simulink model "masseRessort"  (R2014b)
settings: Solver=ode45  StartTime=t0  StopTime=tf  MaxStep=max_step  MinStep=min_step  RelTol=tol
StopFcn:
  | save(wSaveFileName,wSwitchOutputName,wMatlabOutputName)
values from neighbouring files (symbols this model uses):
  b = bs(j)    [masseRessortDataDictionnary.m]    (also in masseRessortDataPost.m)
  b2 = 0    [masseRessortDataDictionnary.m]
  g = 9.8    [masseRessortDataDictionnary.m]
  k1 = 1    [masseRessortDataDictionnary.m]
  k2 = k2s(i)    [masseRessortDataDictionnary.m]    (also in masseRessortDataPost.m)
  m = 1    [masseRessortDataDictionnary.m]
  v0 = -3    [masseRessortDataDictionnary.m]
  x0 = 2    [masseRessortDataDictionnary.m]
  x1 = 1    [masseRessortDataDictionnary.m]
settings Model: Creator=Zangdaarr  LastModifiedBy=Zangdaarr
settings OptimizationCC: InlineParams=on  InlineInvariantSignals=on  EfficientFloat2IntCast=on

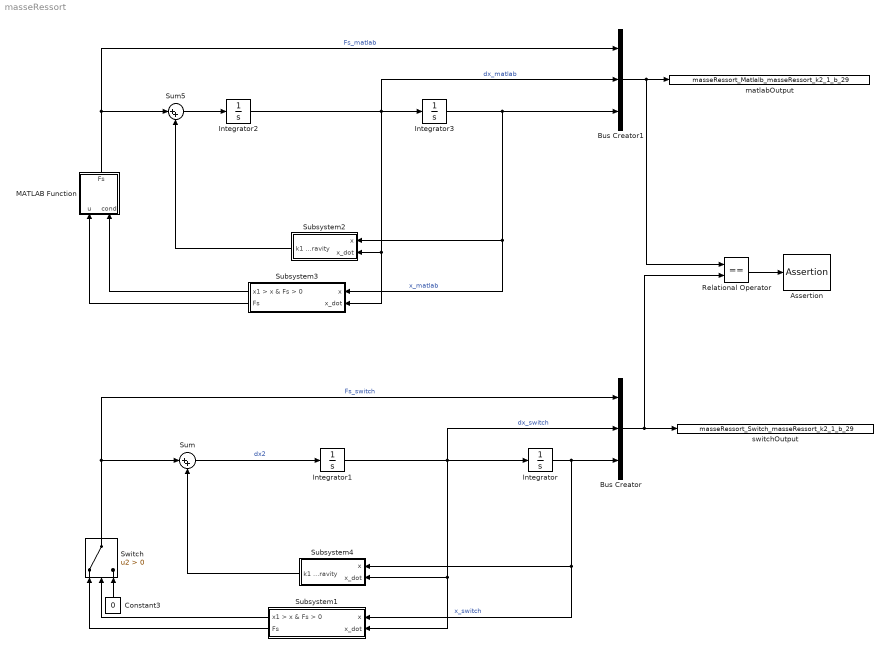
== system masseRessort ==
  Assertion : Assertion
  Bus Creator : BusCreator  Inputs=3
  Bus Creator1 : BusCreator  Inputs=3
  Constant3 : Constant  Value=0
  Integrator : Integrator  InitialCondition=x0
  Integrator1 : Integrator  InitialCondition=v0
  Integrator2 : Integrator  InitialCondition=v0
  Integrator3 : Integrator  InitialCondition=x0
  MATLAB Function : MATLAB Function  TreatAsAtomicUnit=on
  Relational Operator : RelationalOperator  Operator===  OutDataTypeStr=boolean
  Subsystem1 : Subsystem
  Subsystem2 : Subsystem
  Subsystem3 : Subsystem
  Subsystem4 : Subsystem
  Sum : Sum  Inputs=|++
  Sum5 : Sum  Inputs=|++
  Switch : Switch  Criteria=u2 > Threshold
  matlabOutput : ToWorkspace  VariableName=masseRessort_Matlalb_masseRessort_k2_1_b_29  SaveFormat=Timeseries  SampleTime=-1
  switchOutput : ToWorkspace  VariableName=masseRessort_Switch_masseRessort_k2_1_b_29  SaveFormat=Timeseries  SampleTime=-1
  wires:
  Integrator/1 -> Subsystem4/1(x), Subsystem1/1(x), Bus Creator/3  "x_switch"
  Bus Creator/1 -> Relational Operator/2, switchOutput/1
  Bus Creator1/1 -> Relational Operator/1, matlabOutput/1
  Sum/1 -> Integrator1/1  "dx2"
  Integrator1/1 -> Bus Creator/2, Subsystem4/2(x_dot), Subsystem1/2(x_dot), Integrator/1  "dx_switch"
  Subsystem1/1(x1 > x & Fs > 0) -> Switch/2
  Switch/1 -> Sum/1, Bus Creator/1  "Fs_switch"
  Subsystem2/1(k1 + gravity) -> Sum5/2
  Sum5/1 -> Integrator2/1
  Integrator2/1 -> Subsystem3/2(x_dot), Subsystem2/2(x_dot), Bus Creator1/2, Integrator3/1  "dx_matlab"
  Integrator3/1 -> Subsystem3/1(x), Subsystem2/1(x), Bus Creator1/3  "x_matlab"
  MATLAB Function/1(Fs) -> Bus Creator1/1, Sum5/1  "Fs_matlab"
  Subsystem1/2(Fs) -> Switch/1
  Constant3/1 -> Switch/3
  Subsystem3/1(x1 > x & Fs > 0) -> MATLAB Function/2(cond)
  Subsystem3/2(Fs) -> MATLAB Function/1(u)
  Subsystem4/1(k1 + gravity) -> Sum/2
  Relational Operator/1 -> Assertion/1

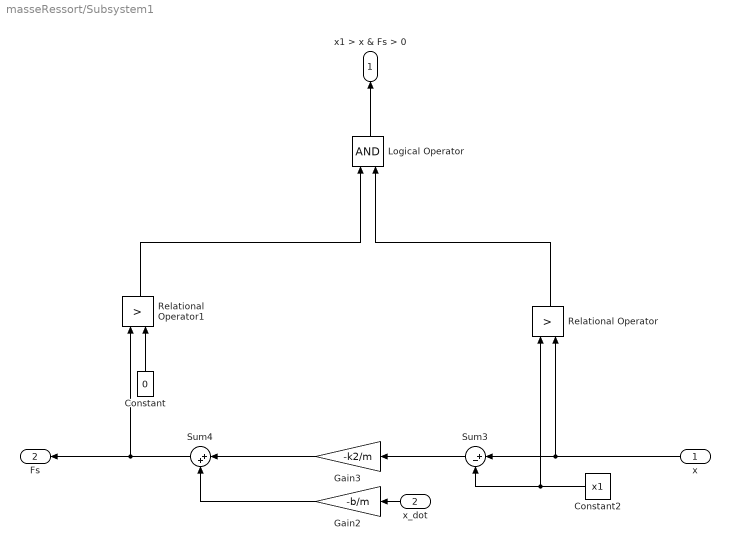
== system masseRessort/Subsystem1 ==
  x : Inport
  x_dot : Inport  Port=2
  Constant : Constant  Value=0
  Constant2 : Constant  Value=x1
  Gain2 : Gain  Gain=-b/m
  Gain3 : Gain  Gain=-k2/m
  Logical Operator : Logic  AllPortsSameDT=off  OutDataTypeStr=boolean
  Relational Operator : RelationalOperator  Operator=>  OutDataTypeStr=boolean
  Relational Operator1 : RelationalOperator  Operator=>  OutDataTypeStr=boolean
  Sum3 : Sum  Inputs=|+-
  Sum4 : Sum  Inputs=|++
  x1 > x & Fs > 0 : Outport
  Fs : Outport  Port=2
  wires:
  Sum3/1 -> Gain3/1
  Constant2/1 -> Sum3/2, Relational Operator/1
  Gain3/1 -> Sum4/1
  Gain2/1 -> Sum4/2
  x_dot/1 -> Gain2/1
  x/1 -> Relational Operator/2, Sum3/1
  Sum4/1 -> Relational Operator1/1, Fs/1
  Constant/1 -> Relational Operator1/2
  Relational Operator1/1 -> Logical Operator/1
  Relational Operator/1 -> Logical Operator/2
  Logical Operator/1 -> x1 > x & Fs > 0/1

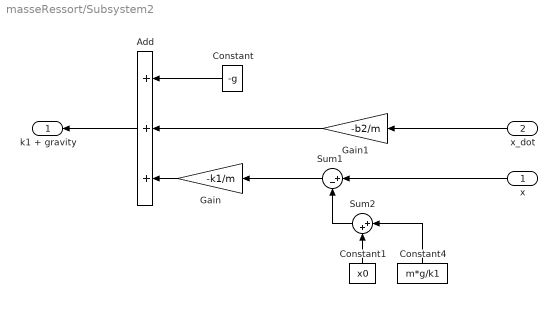
== system masseRessort/Subsystem2 ==
  x : Inport
  x_dot : Inport  Port=2
  Add : Sum  Inputs=+++
  Constant : Constant  Value=-g
  Constant1 : Constant  Value=x0
  Constant4 : Constant  Value=m*g/k1
  Gain : Gain  Gain=-k1/m
  Gain1 : Gain  Gain=-b2/m
  Sum1 : Sum  Inputs=|+-
  Sum2 : Sum  Inputs=|++
  k1 + gravity : Outport
  wires:
  Sum2/1 -> Sum1/2
  Constant4/1 -> Sum2/1
  Constant1/1 -> Sum2/2
  Constant/1 -> Add/1
  Sum1/1 -> Gain/1
  Add/1 -> k1 + gravity/1
  x/1 -> Sum1/1
  Gain1/1 -> Add/2
  Gain/1 -> Add/3
  x_dot/1 -> Gain1/1

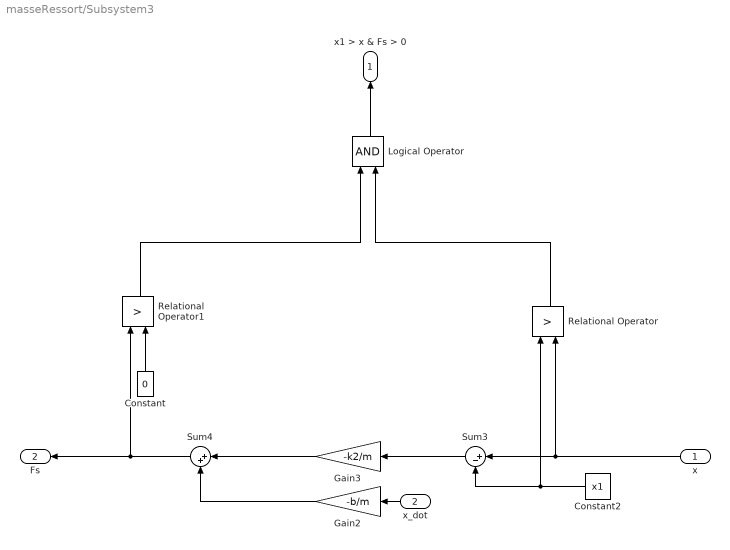
== system masseRessort/Subsystem3 ==
  x : Inport
  x_dot : Inport  Port=2
  Constant : Constant  Value=0
  Constant2 : Constant  Value=x1
  Gain2 : Gain  Gain=-b/m
  Gain3 : Gain  Gain=-k2/m
  Logical Operator : Logic  AllPortsSameDT=off  OutDataTypeStr=boolean
  Relational Operator : RelationalOperator  Operator=>  OutDataTypeStr=boolean
  Relational Operator1 : RelationalOperator  Operator=>  OutDataTypeStr=boolean
  Sum3 : Sum  Inputs=|+-
  Sum4 : Sum  Inputs=|++
  x1 > x & Fs > 0 : Outport
  Fs : Outport  Port=2
  wires:
  Logical Operator/1 -> x1 > x & Fs > 0/1
  Relational Operator/1 -> Logical Operator/2
  Relational Operator1/1 -> Logical Operator/1
  Constant/1 -> Relational Operator1/2
  Sum4/1 -> Fs/1, Relational Operator1/1
  x/1 -> Sum3/1, Relational Operator/2
  x_dot/1 -> Gain2/1
  Gain2/1 -> Sum4/2
  Gain3/1 -> Sum4/1
  Constant2/1 -> Relational Operator/1, Sum3/2
  Sum3/1 -> Gain3/1

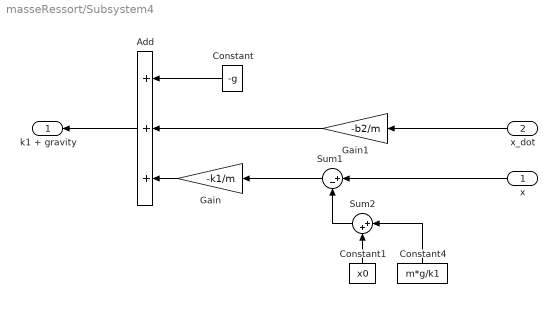
== system masseRessort/Subsystem4 ==
  x : Inport
  x_dot : Inport  Port=2
  Add : Sum  Inputs=+++
  Constant : Constant  Value=-g
  Constant1 : Constant  Value=x0
  Constant4 : Constant  Value=m*g/k1
  Gain : Gain  Gain=-k1/m
  Gain1 : Gain  Gain=-b2/m
  Sum1 : Sum  Inputs=|+-
  Sum2 : Sum  Inputs=|++
  k1 + gravity : Outport
  wires:
  x_dot/1 -> Gain1/1
  Gain/1 -> Add/3
  Gain1/1 -> Add/2
  x/1 -> Sum1/1
  Add/1 -> k1 + gravity/1
  Sum1/1 -> Gain/1
  Constant/1 -> Add/1
  Constant1/1 -> Sum2/2
  Constant4/1 -> Sum2/1
  Sum2/1 -> Sum1/2

== matlab function masseRessort/MATLAB Function ==
  data: u input; cond input; Fs output
function Fs = fcn(u,cond)
%#codegen

if (cond > 0)
    Fs = u;
else
    Fs = 0;
end
